simulink model "PV_MODEL"  (R2024b)
settings: Solver=ode23t  StartTime=0.0  StopTime=2.4  FixedStep=1e-6  RelTol=1e-3
libraries: spsSeriesRLCBranchLib x12, spsFirstOrderFilterLib x9, spsIGBTDiodeLib x7, slpidlib x5, simulink x5, spsThreePhaseVIMeasurementLib x2, spsabctodq0Lib x2, spsAlphaBetaZerotodq0Lib x1, spsDiodeLib x1, spsPVArrayLib x1, spsPower3phInstantaneousLib x1, spsThreePhaseSourceLib x1
settings Model: Creator=Baymax  LastModifiedBy=Baymax

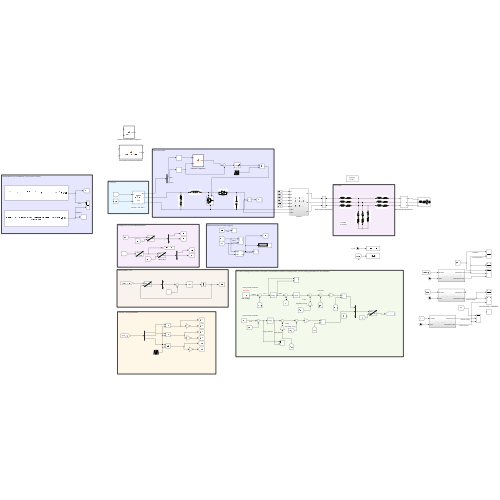
[thumbnail: Simulink's stored preview of the top-level diagram]
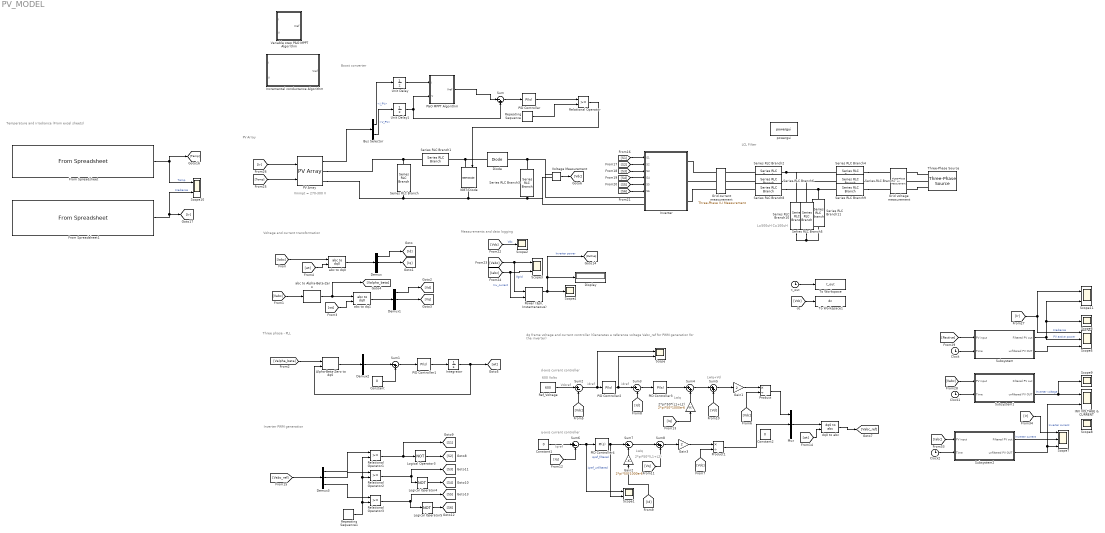
== system PV_MODEL ==
  note: Measurements and data logging
  note: Vmmpt = 270-300 V
  note: PV Array
  note: Boost converter
  note: L=500uH
      | C=100uH
  note: LCL Filter
  note: Inverter PWM generation
  note: dq frame voltage and current controller (Generates a reference voltage Vabc_ref for PWM generation for the inverter)
  note: Three phase - PLL
  note: Voltage and current transformation
  note: d-axis current controller
  note: LwIq+Vd
  note: 600 Volts
  note: 2*pi*50*(L1+L2)
  note: Vdcref
  note: idref
  note: q-axis current controller
  note: LwIq
  note: Iqref
  note: LwIq
  note: idref
  note: Temperature and irradiance (From excel sheets)
  2*pi*50*(L1+L2) : Gain  Gain=2*pi*50*1000e-6
  Alpha-Beta-Zero to dq0 : spsAlphaBetaZerotodq0Lib/Alpha-Beta-Zero to dq0  Alignment=90 degrees behind phase A axis
  Bus Selector : BusSelector  OutputSignals=I_PV,V_PV
  Clock : Clock
  Clock1 : Clock
  Clock2 : Clock
  Constant : Constant  Value=0
  Constant1 : Constant  Value=0
  Constant2 : Constant  Value=0
  Demux{,1..3} (4 alike) : Demux  Outputs=3
  Diode : spsDiodeLib/Diode  Ron=0.001  Lon=0  Vf=0.8  IC=0  UseSnubber=0  Rs=500  Cs=250e-9  Measurements=off
  Display : Display
  From Spreadsheet : FromSpreadsheet  FileName=C:\Users\Baymax\Desktop\Mr.Usamah\Profiles\granular\temperature_profile.xlsx  SheetName=temperature_profile  Range=A2:B2002
  From Spreadsheet1 : FromSpreadsheet  FileName=C:\Users\Baymax\Desktop\Mr.Usamah\Profiles\granular\Irradiance_profile_granular.xlsx  SheetName=irradiance_data  Range=A2:B2002
  Gain1 : Gain  Gain=2
  Gain2 : Gain  Gain=2*pi*50*1000e-6
  Gain3 : Gain  Gain=2
  Grid current measurement : spsThreePhaseVIMeasurementLib/Three-Phase V-I Measurement  VoltageMeasurement=no  SetLabelV=off  LabelV=Vabc  Vpu=off  VpuLL=off  CurrentMeasurement=yes  SetLabelI=on  LabelI=Iabc  Ipu=off  Pbase=100e6  Vbase=500e3  OutputType=Complex  PhasorSimulation=off  PSBequivalent=0
  Grid voltage measurement : spsThreePhaseVIMeasurementLib/Three-Phase V-I Measurement  VoltageMeasurement=phase-to-ground  SetLabelV=on  LabelV=Vabc  Vpu=off  VpuLL=off  CurrentMeasurement=no  SetLabelI=on  LabelI=Iabc  Ipu=off  Pbase=100e6  Vbase=500e3  OutputType=Complex  PhasorSimulation=off  PSBequivalent=0
  IGBT/Diode : spsIGBTDiodeLib/IGBT//Diode  Ron=1e-3  Rs=1e5  Cs=inf  Measurements=off
  INV VOLTAGE & CURRENT : Scope  NumInputPorts=2
  Incremental conductance Algorithm : MATLAB Function  TreatAsAtomicUnit=on
  Integrator : Integrator
  "Inverter " : Subsystem
  Logical Operator3 : Logic  Operator=NOT  IconShape=distinctive  AllPortsSameDT=off  OutDataTypeStr=boolean
  Logical Operator4 : Logic  Operator=NOT  IconShape=distinctive  AllPortsSameDT=off  OutDataTypeStr=boolean
  Logical Operator5 : Logic  Operator=NOT  IconShape=distinctive  AllPortsSameDT=off  OutDataTypeStr=boolean
  Mux : Mux  Inputs=3
  P&O MPPT Algorithm : MATLAB Function  TreatAsAtomicUnit=on
  PID Controller : slpidlib/PID Controller  Controller=PI  Form=Parallel  TimeDomain=Continuous-time  UseExternalTs=off  SampleTime=-1  IntegratorMethod=Forward Euler  FilterMethod=Forward Euler  ControllerParametersSource=internal  P=0.05  I=0.01  UseKiTs=off  D=0  UseExternalDerivativeSource=off  N=100  UseFilter=on  TunerSelectOption=Transfer Function Based (PID Tuner App)  InitialConditionSource=internal  InitialConditionForIntegrator=0  InitialConditionForFilter=0  DifferentiatorICPrevScaledInput=0  ExternalReset=none  TrackingMode=off  Kt=1  LimitOutput=on  SatLimitsSource=internal  UpperSaturationLimit=0.95  LowerSaturationLimit=0  LinearizeAsGain=on  AntiWindupMode=none  Kb=1  LimitIntegrator=off  UpperIntegratorSaturationLimit=inf  LowerIntegratorSaturationLimit=-inf  POutMin=[]  POutMax=[]  IOutMin=[]  IOutMax=[]  DOutMin=[]  DOutMax=[]  NOutMin=[]  NOutMax=[]  SumOutMin=[]  SumOutMax=[]  SaturationOutMin=[]  SaturationOutMax=[]  PParamMin=[]  PParamMax=[]  IParamMin=[]  IParamMax=[]  DParamMin=[]  DParamMax=[]  NParamMin=[]  NParamMax=[]  KbParamMin=[]  KbParamMax=[]  KtParamMin=[]  KtParamMax=[]  KbOutMin=[]  KbOutMax=[]  KtOutMin=[]  KtOutMax=[]  IntegratorOutMin=[]  IntegratorOutMax=[]  FilterOutMin=[]  FilterOutMax=[]  SumI1OutMin=[]  SumI1OutMax=[]  SumI2OutMin=[]  SumI2OutMax=[]  SumI3OutMin=[]  SumI3OutMax=[]  SumI4OutMin=[]  SumI4OutMax=[]  SumDOutMin=[]  SumDOutMax=[]  DifferentiatorOutMin=[]  DifferentiatorOutMax=[]  FilterDiffOutCoefMin=[]  FilterDiffOutCoefMax=[]  ReciprocalOutMin=[]  ReciprocalOutMax=[]  SumDenOutMin=[]  SumDenOutMax=[]  SumNumOutMin=[]  SumNumOutMax=[]  DivideOutMin=[]  DivideOutMax=[]  UdiffTsProdOutMin=[]  UdiffTsProdOutMax=[]  NTsProdOutMin=[]  NTsProdOutMax=[]  UintegralTsProdOutMin=[]  UintegralTsProdOutMax=[]  UngainTsProdOutMin=[]  UngainTsProdOutMax=[]  ClampingZeroOutDataTypeStr=Inherit: Inherit via back propagation  ClampingZeroOutMin=[]  ClampingZeroOutMax=[]  FilterDenConstantOutDataTypeStr=Inherit: Inherit via back propagation  FilterDenConstantOutMin=[]  FilterDenConstantOutMax=[]  PCopyOutDataTypeStr=Inherit: Inherit via back propagation  PCopyOutMin=[]  PCopyOutMax=[]  NCopyOutDataTypeStr=Inherit: Inherit via back propagation  NCopyOutMin=[]  NCopyOutMax=[]  IntegratorContinuousStateAttributes=''  IntegratorStateMustResolveToSignalObject=off  IntegratorRTWStateStorageClass=Auto  FilterContinuousStateAttributes=''  FilterStateMustResolveToSignalObject=off  FilterRTWStateStorageClass=Auto  ParallelPVariant=InternalParameters  IdealPVariant=Disabled  IVariant=InternalParameters  DVariant=Disabled  IntegratorVariant=Continuous  SatVariant=Enabled  AWVariant=Passthrough  PCopyVariant=Disabled  TRVariant=Disabled  FdbkBlocksVariant=Forward  IdealPFdbkVariant=Disabled  SatFdbkVariant=Disabled  DerivativeFilterVariant=Disabled  NVariant=Disabled  NCopyVariant=Disabled_SignalSpec  FilterICVariant=Disabled  IntegratorICVariant=InternalICs  ExternalResetVariant=Disabled  TRSumVariant=Passthrough  SumFdbkVariant=Disabled  SumVariant=Sum_PI  TsampFilterVariant=InternalTs  TsampNgainVariant=Passthrough  TsampIntegralVariant=Disabled_SignalSpec  ExternalSaturationOutDataTypeStr=Inherit: Same as second input  DerivativeSourceVariant=Disabled  PreIntVariant=InternalPreInt
  PID Controller1 : slpidlib/PID Controller  Controller=PI  Form=Parallel  TimeDomain=Continuous-time  UseExternalTs=off  SampleTime=-1  IntegratorMethod=Forward Euler  FilterMethod=Forward Euler  ControllerParametersSource=internal  P=10  I=50000  UseKiTs=off  D=0  UseExternalDerivativeSource=off  N=100  UseFilter=on  TunerSelectOption=Transfer Function Based (PID Tuner App)  InitialConditionSource=internal  InitialConditionForIntegrator=0  InitialConditionForFilter=0  DifferentiatorICPrevScaledInput=0  ExternalReset=none  TrackingMode=off  Kt=1  LimitOutput=off  SatLimitsSource=internal  UpperSaturationLimit=inf  LowerSaturationLimit=-inf  LinearizeAsGain=on  AntiWindupMode=none  Kb=1  LimitIntegrator=off  UpperIntegratorSaturationLimit=inf  LowerIntegratorSaturationLimit=-inf  POutMin=[]  POutMax=[]  IOutMin=[]  IOutMax=[]  DOutMin=[]  DOutMax=[]  NOutMin=[]  NOutMax=[]  SumOutMin=[]  SumOutMax=[]  SaturationOutMin=[]  SaturationOutMax=[]  PParamMin=[]  PParamMax=[]  IParamMin=[]  IParamMax=[]  DParamMin=[]  DParamMax=[]  NParamMin=[]  NParamMax=[]  KbParamMin=[]  KbParamMax=[]  KtParamMin=[]  KtParamMax=[]  KbOutMin=[]  KbOutMax=[]  KtOutMin=[]  KtOutMax=[]  IntegratorOutMin=[]  IntegratorOutMax=[]  FilterOutMin=[]  FilterOutMax=[]  SumI1OutMin=[]  SumI1OutMax=[]  SumI2OutMin=[]  SumI2OutMax=[]  SumI3OutMin=[]  SumI3OutMax=[]  SumI4OutMin=[]  SumI4OutMax=[]  SumDOutMin=[]  SumDOutMax=[]  DifferentiatorOutMin=[]  DifferentiatorOutMax=[]  FilterDiffOutCoefMin=[]  FilterDiffOutCoefMax=[]  ReciprocalOutMin=[]  ReciprocalOutMax=[]  SumDenOutMin=[]  SumDenOutMax=[]  SumNumOutMin=[]  SumNumOutMax=[]  DivideOutMin=[]  DivideOutMax=[]  UdiffTsProdOutMin=[]  UdiffTsProdOutMax=[]  NTsProdOutMin=[]  NTsProdOutMax=[]  UintegralTsProdOutMin=[]  UintegralTsProdOutMax=[]  UngainTsProdOutMin=[]  UngainTsProdOutMax=[]  ClampingZeroOutDataTypeStr=Inherit: Inherit via back propagation  ClampingZeroOutMin=[]  ClampingZeroOutMax=[]  FilterDenConstantOutDataTypeStr=Inherit: Inherit via back propagation  FilterDenConstantOutMin=[]  FilterDenConstantOutMax=[]  PCopyOutDataTypeStr=Inherit: Inherit via back propagation  PCopyOutMin=[]  PCopyOutMax=[]  NCopyOutDataTypeStr=Inherit: Inherit via back propagation  NCopyOutMin=[]  NCopyOutMax=[]  IntegratorContinuousStateAttributes=''  IntegratorStateMustResolveToSignalObject=off  IntegratorRTWStateStorageClass=Auto  FilterContinuousStateAttributes=''  FilterStateMustResolveToSignalObject=off  FilterRTWStateStorageClass=Auto  ParallelPVariant=InternalParameters  IdealPVariant=Disabled  IVariant=InternalParameters  DVariant=Disabled  IntegratorVariant=Continuous  SatVariant=Disabled  AWVariant=Passthrough  PCopyVariant=Disabled  TRVariant=Disabled  FdbkBlocksVariant=Forward  IdealPFdbkVariant=Disabled  SatFdbkVariant=Disabled  DerivativeFilterVariant=Disabled  NVariant=Disabled  NCopyVariant=Disabled_SignalSpec  FilterICVariant=Disabled  IntegratorICVariant=InternalICs  ExternalResetVariant=Disabled  TRSumVariant=Passthrough  SumFdbkVariant=Disabled  SumVariant=Sum_PI  TsampFilterVariant=InternalTs  TsampNgainVariant=Passthrough  TsampIntegralVariant=Disabled_SignalSpec  ExternalSaturationOutDataTypeStr=Inherit: Same as second input  DerivativeSourceVariant=Disabled  PreIntVariant=InternalPreInt
  PID Controller2 : slpidlib/PID Controller  Controller=PI  Form=Parallel  TimeDomain=Continuous-time  UseExternalTs=off  SampleTime=-1  IntegratorMethod=Forward Euler  FilterMethod=Forward Euler  ControllerParametersSource=internal  P=0.25  I=300  UseKiTs=off  D=0  UseExternalDerivativeSource=off  N=100  UseFilter=on  TunerSelectOption=Transfer Function Based (PID Tuner App)  InitialConditionSource=internal  InitialConditionForIntegrator=0  InitialConditionForFilter=0  DifferentiatorICPrevScaledInput=0  ExternalReset=none  TrackingMode=off  Kt=1  LimitOutput=off  SatLimitsSource=internal  UpperSaturationLimit=inf  LowerSaturationLimit=-inf  LinearizeAsGain=on  AntiWindupMode=none  Kb=1  LimitIntegrator=off  UpperIntegratorSaturationLimit=inf  LowerIntegratorSaturationLimit=-inf  POutMin=[]  POutMax=[]  IOutMin=[]  IOutMax=[]  DOutMin=[]  DOutMax=[]  NOutMin=[]  NOutMax=[]  SumOutMin=[]  SumOutMax=[]  SaturationOutMin=[]  SaturationOutMax=[]  PParamMin=[]  PParamMax=[]  IParamMin=[]  IParamMax=[]  DParamMin=[]  DParamMax=[]  NParamMin=[]  NParamMax=[]  KbParamMin=[]  KbParamMax=[]  KtParamMin=[]  KtParamMax=[]  KbOutMin=[]  KbOutMax=[]  KtOutMin=[]  KtOutMax=[]  IntegratorOutMin=[]  IntegratorOutMax=[]  FilterOutMin=[]  FilterOutMax=[]  SumI1OutMin=[]  SumI1OutMax=[]  SumI2OutMin=[]  SumI2OutMax=[]  SumI3OutMin=[]  SumI3OutMax=[]  SumI4OutMin=[]  SumI4OutMax=[]  SumDOutMin=[]  SumDOutMax=[]  DifferentiatorOutMin=[]  DifferentiatorOutMax=[]  FilterDiffOutCoefMin=[]  FilterDiffOutCoefMax=[]  ReciprocalOutMin=[]  ReciprocalOutMax=[]  SumDenOutMin=[]  SumDenOutMax=[]  SumNumOutMin=[]  SumNumOutMax=[]  DivideOutMin=[]  DivideOutMax=[]  UdiffTsProdOutMin=[]  UdiffTsProdOutMax=[]  NTsProdOutMin=[]  NTsProdOutMax=[]  UintegralTsProdOutMin=[]  UintegralTsProdOutMax=[]  UngainTsProdOutMin=[]  UngainTsProdOutMax=[]  ClampingZeroOutDataTypeStr=Inherit: Inherit via back propagation  ClampingZeroOutMin=[]  ClampingZeroOutMax=[]  FilterDenConstantOutDataTypeStr=Inherit: Inherit via back propagation  FilterDenConstantOutMin=[]  FilterDenConstantOutMax=[]  PCopyOutDataTypeStr=Inherit: Inherit via back propagation  PCopyOutMin=[]  PCopyOutMax=[]  NCopyOutDataTypeStr=Inherit: Inherit via back propagation  NCopyOutMin=[]  NCopyOutMax=[]  IntegratorContinuousStateAttributes=''  IntegratorStateMustResolveToSignalObject=off  IntegratorRTWStateStorageClass=Auto  FilterContinuousStateAttributes=''  FilterStateMustResolveToSignalObject=off  FilterRTWStateStorageClass=Auto  ParallelPVariant=InternalParameters  IdealPVariant=Disabled  IVariant=InternalParameters  DVariant=Disabled  IntegratorVariant=Continuous  SatVariant=Disabled  AWVariant=Passthrough  PCopyVariant=Disabled  TRVariant=Disabled  FdbkBlocksVariant=Forward  IdealPFdbkVariant=Disabled  SatFdbkVariant=Disabled  DerivativeFilterVariant=Disabled  NVariant=Disabled  NCopyVariant=Disabled_SignalSpec  FilterICVariant=Disabled  IntegratorICVariant=InternalICs  ExternalResetVariant=Disabled  TRSumVariant=Passthrough  SumFdbkVariant=Disabled  SumVariant=Sum_PI  TsampFilterVariant=InternalTs  TsampNgainVariant=Passthrough  TsampIntegralVariant=Disabled_SignalSpec  ExternalSaturationOutDataTypeStr=Inherit: Same as second input  DerivativeSourceVariant=Disabled  PreIntVariant=InternalPreInt
  PID Controller3 : slpidlib/PID Controller  Controller=PI  Form=Parallel  TimeDomain=Continuous-time  UseExternalTs=off  SampleTime=-1  IntegratorMethod=Forward Euler  FilterMethod=Forward Euler  ControllerParametersSource=internal  P=10  I=20  UseKiTs=off  D=0  UseExternalDerivativeSource=off  N=100  UseFilter=on  TunerSelectOption=Transfer Function Based (PID Tuner App)  InitialConditionSource=internal  InitialConditionForIntegrator=0  InitialConditionForFilter=0  DifferentiatorICPrevScaledInput=0  ExternalReset=none  TrackingMode=off  Kt=1  LimitOutput=off  SatLimitsSource=internal  UpperSaturationLimit=inf  LowerSaturationLimit=-inf  LinearizeAsGain=on  AntiWindupMode=none  Kb=1  LimitIntegrator=off  UpperIntegratorSaturationLimit=inf  LowerIntegratorSaturationLimit=-inf  POutMin=[]  POutMax=[]  IOutMin=[]  IOutMax=[]  DOutMin=[]  DOutMax=[]  NOutMin=[]  NOutMax=[]  SumOutMin=[]  SumOutMax=[]  SaturationOutMin=[]  SaturationOutMax=[]  PParamMin=[]  PParamMax=[]  IParamMin=[]  IParamMax=[]  DParamMin=[]  DParamMax=[]  NParamMin=[]  NParamMax=[]  KbParamMin=[]  KbParamMax=[]  KtParamMin=[]  KtParamMax=[]  KbOutMin=[]  KbOutMax=[]  KtOutMin=[]  KtOutMax=[]  IntegratorOutMin=[]  IntegratorOutMax=[]  FilterOutMin=[]  FilterOutMax=[]  SumI1OutMin=[]  SumI1OutMax=[]  SumI2OutMin=[]  SumI2OutMax=[]  SumI3OutMin=[]  SumI3OutMax=[]  SumI4OutMin=[]  SumI4OutMax=[]  SumDOutMin=[]  SumDOutMax=[]  DifferentiatorOutMin=[]  DifferentiatorOutMax=[]  FilterDiffOutCoefMin=[]  FilterDiffOutCoefMax=[]  ReciprocalOutMin=[]  ReciprocalOutMax=[]  SumDenOutMin=[]  SumDenOutMax=[]  SumNumOutMin=[]  SumNumOutMax=[]  DivideOutMin=[]  DivideOutMax=[]  UdiffTsProdOutMin=[]  UdiffTsProdOutMax=[]  NTsProdOutMin=[]  NTsProdOutMax=[]  UintegralTsProdOutMin=[]  UintegralTsProdOutMax=[]  UngainTsProdOutMin=[]  UngainTsProdOutMax=[]  ClampingZeroOutDataTypeStr=Inherit: Inherit via back propagation  ClampingZeroOutMin=[]  ClampingZeroOutMax=[]  FilterDenConstantOutDataTypeStr=Inherit: Inherit via back propagation  FilterDenConstantOutMin=[]  FilterDenConstantOutMax=[]  PCopyOutDataTypeStr=Inherit: Inherit via back propagation  PCopyOutMin=[]  PCopyOutMax=[]  NCopyOutDataTypeStr=Inherit: Inherit via back propagation  NCopyOutMin=[]  NCopyOutMax=[]  IntegratorContinuousStateAttributes=''  IntegratorStateMustResolveToSignalObject=off  IntegratorRTWStateStorageClass=Auto  FilterContinuousStateAttributes=''  FilterStateMustResolveToSignalObject=off  FilterRTWStateStorageClass=Auto  ParallelPVariant=InternalParameters  IdealPVariant=Disabled  IVariant=InternalParameters  DVariant=Disabled  IntegratorVariant=Continuous  SatVariant=Disabled  AWVariant=Passthrough  PCopyVariant=Disabled  TRVariant=Disabled  FdbkBlocksVariant=Forward  IdealPFdbkVariant=Disabled  SatFdbkVariant=Disabled  DerivativeFilterVariant=Disabled  NVariant=Disabled  NCopyVariant=Disabled_SignalSpec  FilterICVariant=Disabled  IntegratorICVariant=InternalICs  ExternalResetVariant=Disabled  TRSumVariant=Passthrough  SumFdbkVariant=Disabled  SumVariant=Sum_PI  TsampFilterVariant=InternalTs  TsampNgainVariant=Passthrough  TsampIntegralVariant=Disabled_SignalSpec  ExternalSaturationOutDataTypeStr=Inherit: Same as second input  DerivativeSourceVariant=Disabled  PreIntVariant=InternalPreInt
  PID Controller4 : slpidlib/PID Controller  Controller=PI  Form=Parallel  TimeDomain=Continuous-time  UseExternalTs=off  SampleTime=-1  IntegratorMethod=Forward Euler  FilterMethod=Forward Euler  ControllerParametersSource=internal  P=10  I=20  UseKiTs=off  D=0  UseExternalDerivativeSource=off  N=100  UseFilter=on  TunerSelectOption=Transfer Function Based (PID Tuner App)  InitialConditionSource=internal  InitialConditionForIntegrator=0  InitialConditionForFilter=0  DifferentiatorICPrevScaledInput=0  ExternalReset=none  TrackingMode=off  Kt=1  LimitOutput=off  SatLimitsSource=internal  UpperSaturationLimit=inf  LowerSaturationLimit=-inf  LinearizeAsGain=on  AntiWindupMode=none  Kb=1  LimitIntegrator=off  UpperIntegratorSaturationLimit=inf  LowerIntegratorSaturationLimit=-inf  POutMin=[]  POutMax=[]  IOutMin=[]  IOutMax=[]  DOutMin=[]  DOutMax=[]  NOutMin=[]  NOutMax=[]  SumOutMin=[]  SumOutMax=[]  SaturationOutMin=[]  SaturationOutMax=[]  PParamMin=[]  PParamMax=[]  IParamMin=[]  IParamMax=[]  DParamMin=[]  DParamMax=[]  NParamMin=[]  NParamMax=[]  KbParamMin=[]  KbParamMax=[]  KtParamMin=[]  KtParamMax=[]  KbOutMin=[]  KbOutMax=[]  KtOutMin=[]  KtOutMax=[]  IntegratorOutMin=[]  IntegratorOutMax=[]  FilterOutMin=[]  FilterOutMax=[]  SumI1OutMin=[]  SumI1OutMax=[]  SumI2OutMin=[]  SumI2OutMax=[]  SumI3OutMin=[]  SumI3OutMax=[]  SumI4OutMin=[]  SumI4OutMax=[]  SumDOutMin=[]  SumDOutMax=[]  DifferentiatorOutMin=[]  DifferentiatorOutMax=[]  FilterDiffOutCoefMin=[]  FilterDiffOutCoefMax=[]  ReciprocalOutMin=[]  ReciprocalOutMax=[]  SumDenOutMin=[]  SumDenOutMax=[]  SumNumOutMin=[]  SumNumOutMax=[]  DivideOutMin=[]  DivideOutMax=[]  UdiffTsProdOutMin=[]  UdiffTsProdOutMax=[]  NTsProdOutMin=[]  NTsProdOutMax=[]  UintegralTsProdOutMin=[]  UintegralTsProdOutMax=[]  UngainTsProdOutMin=[]  UngainTsProdOutMax=[]  ClampingZeroOutDataTypeStr=Inherit: Inherit via back propagation  ClampingZeroOutMin=[]  ClampingZeroOutMax=[]  FilterDenConstantOutDataTypeStr=Inherit: Inherit via back propagation  FilterDenConstantOutMin=[]  FilterDenConstantOutMax=[]  PCopyOutDataTypeStr=Inherit: Inherit via back propagation  PCopyOutMin=[]  PCopyOutMax=[]  NCopyOutDataTypeStr=Inherit: Inherit via back propagation  NCopyOutMin=[]  NCopyOutMax=[]  IntegratorContinuousStateAttributes=''  IntegratorStateMustResolveToSignalObject=off  IntegratorRTWStateStorageClass=Auto  FilterContinuousStateAttributes=''  FilterStateMustResolveToSignalObject=off  FilterRTWStateStorageClass=Auto  ParallelPVariant=InternalParameters  IdealPVariant=Disabled  IVariant=InternalParameters  DVariant=Disabled  IntegratorVariant=Continuous  SatVariant=Disabled  AWVariant=Passthrough  PCopyVariant=Disabled  TRVariant=Disabled  FdbkBlocksVariant=Forward  IdealPFdbkVariant=Disabled  SatFdbkVariant=Disabled  DerivativeFilterVariant=Disabled  NVariant=Disabled  NCopyVariant=Disabled_SignalSpec  FilterICVariant=Disabled  IntegratorICVariant=InternalICs  ExternalResetVariant=Disabled  TRSumVariant=Passthrough  SumFdbkVariant=Disabled  SumVariant=Sum_PI  TsampFilterVariant=InternalTs  TsampNgainVariant=Passthrough  TsampIntegralVariant=Disabled_SignalSpec  ExternalSaturationOutDataTypeStr=Inherit: Same as second input  DerivativeSourceVariant=Disabled  PreIntVariant=InternalPreInt
  PV Array : spsPVArrayLib/PV Array  Npar=47  Nser=10  PlotType=array @ 1000 W/m2 & specified temperatures  S_vec="[ 1000  500  100 ]"  Temp_C_vec="[ 45 25  ]"  ModuleName=A10Green Technology A10J-M60-220  PlotWhenSelected=off  Pm=219.876  Ncell=60  Voc=36.06  Isc=7.95  Vm=30.12  Im=7.3  beta_Voc_pc=-0.3624  alpha_Isc_pc=0.054805  beta_Voc=-0.13068  alpha_Isc=0.004357  IL=7.9642  I0=2.8692e-10  nI=0.97455  Rsh=106.1817  Rs=0.18964  RobustModel=off  RobustCellTemperature=313.3991  BAL=on  Tc=1e-6  Tfilter=5e-5
  "Power (3ph, Instantaneous)" : spsPower3phInstantaneousLib/Power (3ph, Instantaneous)
  Product : Product  Inputs=*/
  Product1 : Product  Inputs=*/
  Ref_Voltage : Constant  Value=600
  Relational Operator{,1..3} (4 alike) : RelationalOperator  OutDataTypeStr=boolean  RndMeth=Simplest  InputSameDT=off
  Repeating Sequence : simulink/Sources/Repeating Sequence  rep_seq_t=[0 0.0002]  rep_seq_y=[0 1]
  Repeating Sequence1 : simulink/Sources/Repeating Sequence  rep_seq_t=[0 0.00005 0.0001]  rep_seq_y=[-1 1 -1]
  Scope{,1,3,10..11} (5 alike) : Scope  NumInputPorts=2
  Scope{2,4,6,8..9} (5 alike) : Scope
  Scope5 : Scope  NumInputPorts=3
  Scope7 : Scope  NumInputPorts=3
  Series RLC Branch : spsSeriesRLCBranchLib/Series RLC Branch  LConnTagsString=__new0  RConnTagsString=__new0  BranchType=RC  Resistance=1e-3  Inductance=1e-3  SetiL0=off  InitialCurrent=0  Capacitance=1000e-6  Setx0=off  InitialVoltage=0  Measurements=None
  Series RLC Branch1 : spsSeriesRLCBranchLib/Series RLC Branch  LConnTagsString=__new0  RConnTagsString=__new0  BranchType=L  Resistance=1  Inductance=1.45e-3  SetiL0=off  InitialCurrent=0  Capacitance=1e-6  Setx0=off  InitialVoltage=0  Measurements=None
  Series RLC Branch10 : spsSeriesRLCBranchLib/Series RLC Branch  LConnTagsString=__new0  RConnTagsString=__new0  BranchType=RC  Resistance=1e-3  Inductance=1e-3  SetiL0=off  InitialCurrent=0  Capacitance=100e-6  Setx0=off  InitialVoltage=0  Measurements=None
  Series RLC Branch11 : spsSeriesRLCBranchLib/Series RLC Branch  LConnTagsString=__new0  RConnTagsString=__new0  BranchType=RC  Resistance=1e-3  Inductance=1e-3  SetiL0=off  InitialCurrent=0  Capacitance=100e-6  Setx0=off  InitialVoltage=0  Measurements=None
  Series RLC Branch{2,4,6..9} (6 alike) : spsSeriesRLCBranchLib/Series RLC Branch  LConnTagsString=__new0  RConnTagsString=__new0  BranchType=RL  Resistance=1e-3  Inductance=500e-6  SetiL0=off  InitialCurrent=0  Capacitance=1e-6  Setx0=off  InitialVoltage=0  Measurements=None
  Series RLC Branch3 : spsSeriesRLCBranchLib/Series RLC Branch  LConnTagsString=__new0  RConnTagsString=__new0  BranchType=C  Resistance=1  Inductance=1e-3  SetiL0=off  InitialCurrent=0  Capacitance=3227e-6  Setx0=off  InitialVoltage=0  Measurements=None
  Series RLC Branch5 : spsSeriesRLCBranchLib/Series RLC Branch  LConnTagsString=__new0  RConnTagsString=__new0  BranchType=RC  Resistance=1e-3  Inductance=1e-3  SetiL0=off  InitialCurrent=0  Capacitance=100e-6  Setx0=off  InitialVoltage=0  Measurements=None
  Subsystem : Subsystem
  Subsystem1 : Subsystem
  Subsystem2 : Subsystem
  Sum : Sum  Inputs=|-+
  Sum1 : Sum  Inputs=|-+
  Sum{2..3,6..7} (4 alike) : Sum  Inputs=|+-
  Sum4 : Sum  Inputs=|++
  Sum5 : Sum  Inputs=|++
  Sum8 : Sum  Inputs=|++
  Three-Phase Source : spsThreePhaseSourceLib/Three-Phase Source  InternalConnection=Yg  VoltagePhases=off  Voltage=400  PhaseAngle=0  Voltage_phases=[25e3 25e3 25e3]/sqrt(3)  PhaseAngles_phases=[0 -120 +120]  Frequency=50  NonIdealSource=on  SpecifyImpedance=off  Resistance=1e-6  Inductance=1e-6  ShortCircuitLevel=100e6  BaseVoltage=400  XRratio=7  BusType=swing  Pref=10e3  Qref=0  Prefabc=[10e3, 10e3, 10e3]  Qrefabc=[0, 0, 0]  Qmin=-inf  Qmax=inf
  To Workspace : ToWorkspace  VariableName=t_out  SampleTime=-1
      settings: Decimation=5
  To Workspace1 : ToWorkspace  VariableName=dc  SampleTime=-1
      settings: Decimation=2
  Unit Delay : UnitDelay  SampleTime=1e-4  HasFrameUpgradeWarning=on
  Unit Delay1 : UnitDelay  SampleTime=1e-4  HasFrameUpgradeWarning=on
  Variable step P&O MPPT Algorithm : MATLAB Function  TreatAsAtomicUnit=on
  Voltage Measurement : spsVoltageMeasurementLib/Voltage Measurement  PhasorSimulation=off  OutputType=Complex  PSBequivalent=0
  abc to Alpha-Beta-Zero : spsabctoAlphaBetaZeroLib/abc to Alpha-Beta-Zero
  abc to dq0 : spsabctodq0Lib/abc to dq0  Alignment=90 degrees behind phase A axis
  abc to dq1 : spsabctodq0Lib/abc to dq0  Alignment=90 degrees behind phase A axis
  dq0 to abc : spsdq0toabcLib/dq0 to abc  Alignment=90 degrees behind phase A axis
  powergui : spspowerguiLib/powergui  Priority=1  SimulationMode=Discrete  SampleTime=1e-6  frequency=60  Iterations=50  frequencyindice=0  Pbase=100e6  ErrMax=1e-4  UnitsV=kV  UnitsW=MW  buscounter=0  FunctionMessages=off  echomessages=off  EnableUseOfTLC=off  CurrentSourceSwitches=off  DisableSnubberDevices=off  DisableRonSwitches=off  DisableVfSwitches=off  DisplayEquations=off  AutomaticDiscreteSolvers=off  SolverType=Tustin/Backward Euler (TBE)  Interpol=off  ExternalGateDelay=off  methode=off  Ts=100  x0status=blocks  SPID=on  SwTol=0  HookPort=off  NonlinearTolerance=1e-4  nMaxIteration=100  ContinueOnMaxIteration=off  RestoreLinks=warning  ResistiveCurrentMeasurement=off  Frange=[0:2:500]  Ylog=off  Xlog=on  ShowGrid=off  save=off  variable=ZData  structure=0  ZoomFFT=off  StartTime=0.0  cycles=1  DisplayStyle=1  fundamental=60  FreqAxis=off  MaxFrequency=1000  frequencyindicesteady=1  RmsSteady=1  display=off
  t_out : Clock
  wires:
  PV Array/1 -> Bus Selector/1
  Bus Selector/1 -> Unit Delay/1  "<I_PV>"
  Bus Selector/2 -> Unit Delay1/1  "<V_PV>"
  Unit Delay1/1 -> P&O MPPT Algorithm/2(V), Sum/2
  Sum/1 -> PID Controller/1
  PID Controller/1 -> Relational Operator/1
  Repeating Sequence/1 -> Relational Operator/2
  Relational Operator/1 -> IGBT/Diode/1
  [Iabc] -> abc to dq0/1
  abc to dq0/1 -> Demux/1
  Demux/1 -> [Id]
  Demux/2 -> [Iq]
  [Vabc] -> abc to Alpha-Beta-Zero/1
  abc to Alpha-Beta-Zero/1 -> [Valpha_beta], abc to dq1/1
  Demux1/2 -> [Vq]
  Demux1/1 -> [Vd]
  abc to dq1/1 -> Demux1/1
  [Valpha_beta] -> Alpha-Beta-Zero to dq0/1
  Alpha-Beta-Zero to dq0/1 -> Demux2/1
  Demux2/2 -> Sum1/1
  Constant/1 -> Sum1/2
  Sum1/1 -> PID Controller1/1
  PID Controller1/1 -> Integrator/1
  Integrator/1 -> [wt], Alpha-Beta-Zero to dq0/2
  [wt] -> abc to dq1/2
  [wt] -> abc to dq0/2
  Gain2/1 -> Sum7/2
  2*pi*50*(L1+L2)/1 -> Sum4/2
  Sum6/1 -> Scope1/1, PID Controller4/1  "iqref_unfiltered"
  [Vq] -> Sum8/2
  PID Controller3/1 -> Sum4/1
  Product/1 -> Mux/1
  Constant1/1 -> Sum6/1
  Mux/1 -> dq0 to abc/1
  Ref_Voltage/1 -> Sum2/1
  Gain3/1 -> Product1/1
  Sum8/1 -> Gain3/1
  PID Controller4/1 -> Sum7/1, Scope1/2  "iqref_filtered"
  Sum4/1 -> Sum5/1
  Sum2/1 -> Scope/1, PID Controller2/1
  Sum3/1 -> PID Controller3/1
  Product1/1 -> Mux/2
  PID Controller2/1 -> Scope/2, Sum3/1
  [Vd] -> Sum5/2
  Sum7/1 -> Sum8/1
  Sum5/1 -> Gain1/1
  Gain1/1 -> Product/1
  Voltage Measurement/1 -> [Vdc]
  [Vdc] -> Sum2/2
  [Vdc] -> Product/2
  [Vdc] -> Product1/2
  [Id] -> Sum3/2
  [Id] -> Gain2/1
  [Iq] -> Sum6/2
  [Iq] -> 2*pi*50*(L1+L2)/1
  [wt] -> dq0 to abc/2
  dq0 to abc/1 -> [Vabc_ref]
  [Vabc_ref] -> Demux3/1
  Demux3/1 -> Relational Operator1/1
  Demux3/2 -> Relational Operator2/1
  Demux3/3 -> Relational Operator3/1
  Repeating Sequence1/1 -> Relational Operator3/2, Relational Operator2/2, Relational Operator1/2
  Relational Operator1/1 -> [S1], Logical Operator3/1
  Logical Operator3/1 -> [S2]
  Relational Operator2/1 -> Logical Operator4/1, [S3]
  Logical Operator4/1 -> [S4]
  Relational Operator3/1 -> Logical Operator5/1, [S5]
  Logical Operator5/1 -> [S6]
  [S1] -> "Inverter "/1(S1)
  [S2] -> "Inverter "/2(S2)
  [S3] -> "Inverter "/3(S3)
  [S4] -> "Inverter "/4(S4)
  [S5] -> "Inverter "/5(S5)
  [S6] -> "Inverter "/6(S6)
  [Vdc] -> Scope2/1  "Vdc"
  [Vabc] -> "Power (3ph, Instantaneous)"/1, Scope3/1  "Vgrid"
  [Iabc] -> "Power (3ph, Instantaneous)"/2, Scope3/2  "Inv_current"
  "Power (3ph, Instantaneous)"/1 -> [Pactive], Display/1, Scope4/1  "Inverter power"
  [Ir] -> PV Array/1
  [Temp] -> PV Array/2
  From Spreadsheet/1 -> [Temp], Scope10/1  "Temp"
  From Spreadsheet1/1 -> Scope10/2, [Ir]  "Irradiance"
  P&O MPPT Algorithm/1(Vref) -> Sum/1
  [Vdc] -> To Workspace1/1
  t_out/1 -> To Workspace/1
  Unit Delay/1 -> P&O MPPT Algorithm/1(I)
  Subsystem/2(unfiltered PV OUT) -> Scope5/3
  Subsystem/1(Filtered PV out) -> Scope11/2, Scope6/1, Scope5/2  "PV active power"
  [Ir] -> Scope5/1, Scope11/1  "Irradiance"
  [Pactive] -> Subsystem/1(PV input)
  Clock/1 -> Subsystem/2(Time)
  Clock1/1 -> Subsystem1/2(Time)
  [Vabc] -> Subsystem1/1(PV input)
  Subsystem1/2(unfiltered PV OUT) -> Scope9/1, INV VOLTAGE & CURRENT/1  "Inverter voltage"
  Subsystem2/2(unfiltered PV OUT) -> INV VOLTAGE & CURRENT/2, Scope7/3  "Inverter current"
  Subsystem2/1(Filtered PV out) -> Scope7/2  "Inverter current"
  [Ir] -> Scope7/1
  [Iabc] -> Subsystem2/1(PV input)
  Clock2/1 -> Subsystem2/2(Time)
  connections:
  Diode/LConn1 -- IGBT/Diode/LConn1 -- Series RLC Branch1/LConn1
  Series RLC Branch1/RConn1 -- PV Array/RConn1 -- Series RLC Branch/LConn1
  Series RLC Branch/RConn1 -- PV Array/RConn2 -- "Inverter "/LConn2 -- Voltage Measurement/LConn2 -- Series RLC Branch3/RConn1 -- IGBT/Diode/RConn1
  Series RLC Branch3/LConn1 -- Voltage Measurement/LConn1 -- "Inverter "/LConn1 -- Diode/RConn1
  Grid current measurement/LConn2 -- "Inverter "/RConn2
  Series RLC Branch2/RConn1 -- Grid current measurement/RConn1
  Series RLC Branch2/LConn1 -- Series RLC Branch10/RConn1 -- Series RLC Branch4/RConn1
  Three-Phase Source/RConn1 -- Grid voltage measurement/LConn1
  Three-Phase Source/RConn2 -- Grid voltage measurement/LConn2
  Three-Phase Source/RConn3 -- Grid voltage measurement/LConn3
  Series RLC Branch4/LConn1 -- Grid voltage measurement/RConn1
  Series RLC Branch6/RConn1 -- Grid current measurement/RConn2
  Series RLC Branch6/LConn1 -- Series RLC Branch5/RConn1 -- Series RLC Branch7/RConn1
  Series RLC Branch7/LConn1 -- Grid voltage measurement/RConn2
  Series RLC Branch8/RConn1 -- Grid current measurement/RConn3
  Series RLC Branch9/LConn1 -- Grid voltage measurement/RConn3
  Series RLC Branch11/RConn1 -- Series RLC Branch9/RConn1 -- Series RLC Branch8/LConn1
  Series RLC Branch11/LConn1 -- Series RLC Branch10/LConn1 -- Series RLC Branch5/LConn1
  Grid current measurement/LConn1 -- "Inverter "/RConn1
  Grid current measurement/LConn3 -- "Inverter "/RConn3

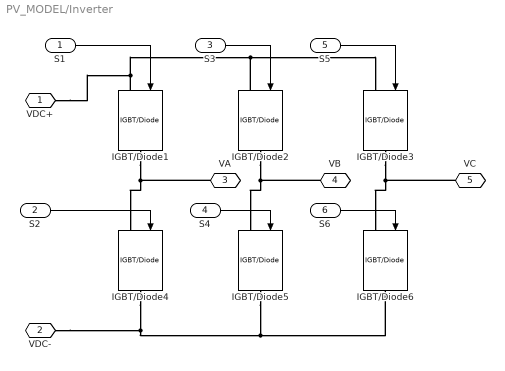
== system PV_MODEL/Inverter  ==
  S1 : Inport
  S2 : Inport  Port=2
  S3 : Inport  Port=3
  S4 : Inport  Port=4
  S5 : Inport  Port=5
  S6 : Inport  Port=6
  IGBT/Diode{1..6} (6 alike) : spsIGBTDiodeLib/IGBT//Diode  Ron=1e-3  Rs=1e5  Cs=inf  Measurements=off
  VDC+ : PMIOPort  Side=Left
  VDC- : PMIOPort  Port=2  Side=Left
  VA : PMIOPort  Port=3  Side=Right
  VB : PMIOPort  Port=4  Side=Right
  VC : PMIOPort  Port=5  Side=Right
  wires:
  S3/1 -> IGBT/Diode2/1
  S2/1 -> IGBT/Diode4/1
  S1/1 -> IGBT/Diode1/1
  S4/1 -> IGBT/Diode5/1
  S6/1 -> IGBT/Diode6/1
  S5/1 -> IGBT/Diode3/1
  connections:
  IGBT/Diode1/LConn1 -- VDC+/RConn1 -- IGBT/Diode2/LConn1 -- IGBT/Diode3/LConn1
  IGBT/Diode2/RConn1 -- VB/RConn1 -- IGBT/Diode5/LConn1
  IGBT/Diode4/RConn1 -- VDC-/RConn1 -- IGBT/Diode6/RConn1 -- IGBT/Diode5/RConn1
  IGBT/Diode1/RConn1 -- VA/RConn1 -- IGBT/Diode4/LConn1
  IGBT/Diode3/RConn1 -- VC/RConn1 -- IGBT/Diode6/LConn1

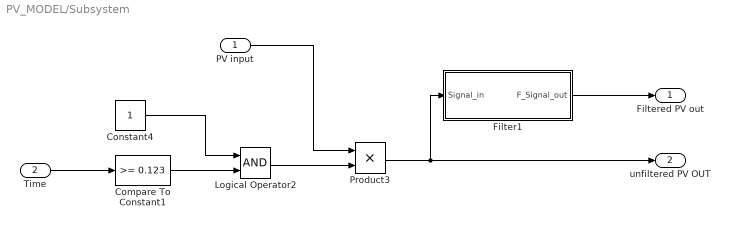
== system PV_MODEL/Subsystem ==
  PV input : Inport
  Time : Inport  Port=2
  Compare To Constant1 : simulink/Logic and Bit Operations/Compare To Constant  relop=>=  const=0.123  OutDataTypeStr=boolean
  Constant4 : Constant
  Filter1 : Subsystem
  Logical Operator2 : Logic  AllPortsSameDT=off  OutDataTypeStr=boolean
  Product3 : Product
  Filtered PV out : Outport
  unfiltered PV OUT : Outport  Port=2
  wires:
  Product3/1 -> unfiltered PV OUT/1, Filter1/1(Signal_in)
  Time/1 -> Compare To Constant1/1
  Constant4/1 -> Logical Operator2/1
  Filter1/1(F_Signal_out) -> Filtered PV out/1
  PV input/1 -> Product3/1
  Logical Operator2/1 -> Product3/2
  Compare To Constant1/1 -> Logical Operator2/2

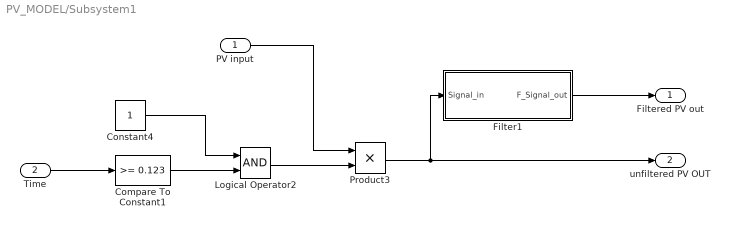
== system PV_MODEL/Subsystem1 ==
  PV input : Inport
  Time : Inport  Port=2
  Compare To Constant1 : simulink/Logic and Bit Operations/Compare To Constant  relop=>=  const=0.123  OutDataTypeStr=boolean
  Constant4 : Constant
  Filter1 : Subsystem
  Logical Operator2 : Logic  AllPortsSameDT=off  OutDataTypeStr=boolean
  Product3 : Product
  Filtered PV out : Outport
  unfiltered PV OUT : Outport  Port=2
  wires:
  Compare To Constant1/1 -> Logical Operator2/2
  Logical Operator2/1 -> Product3/2
  PV input/1 -> Product3/1
  Filter1/1(F_Signal_out) -> Filtered PV out/1
  Constant4/1 -> Logical Operator2/1
  Time/1 -> Compare To Constant1/1
  Product3/1 -> Filter1/1(Signal_in), unfiltered PV OUT/1

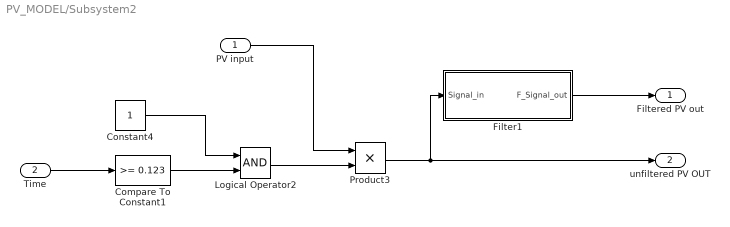
== system PV_MODEL/Subsystem2 ==
  PV input : Inport
  Time : Inport  Port=2
  Compare To Constant1 : simulink/Logic and Bit Operations/Compare To Constant  relop=>=  const=0.123  OutDataTypeStr=boolean
  Constant4 : Constant
  Filter1 : Subsystem
  Logical Operator2 : Logic  AllPortsSameDT=off  OutDataTypeStr=boolean
  Product3 : Product
  Filtered PV out : Outport
  unfiltered PV OUT : Outport  Port=2
  wires:
  Product3/1 -> unfiltered PV OUT/1, Filter1/1(Signal_in)
  Time/1 -> Compare To Constant1/1
  Constant4/1 -> Logical Operator2/1
  Filter1/1(F_Signal_out) -> Filtered PV out/1
  PV input/1 -> Product3/1
  Logical Operator2/1 -> Product3/2
  Compare To Constant1/1 -> Logical Operator2/2

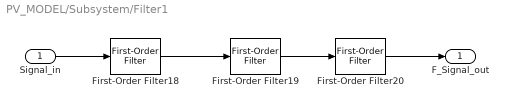
== system PV_MODEL/Subsystem/Filter1 ==
  Signal_in : Inport
  First-Order Filter18 : spsFirstOrderFilterLib/First-Order Filter  FilterType=Lowpass  Tc=1/(2*pi*50)  Ts=0  Initialize=off  Vac_Init=[0, 0, 50]  Vdc_Init=0  PlotResponse=off  FreqRange="[0,  200,  1]"
  First-Order Filter19 : spsFirstOrderFilterLib/First-Order Filter  FilterType=Lowpass  Tc=1/(2*pi*50)  Ts=0  Initialize=off  Vac_Init=[0, 0, 50]  Vdc_Init=0  PlotResponse=off  FreqRange="[0,  200,  1]"
  First-Order Filter20 : spsFirstOrderFilterLib/First-Order Filter  FilterType=Lowpass  Tc=1/(2*pi*50)  Ts=0  Initialize=off  Vac_Init=[0, 0, 50]  Vdc_Init=0  PlotResponse=off  FreqRange="[0,  200,  1]"
  F_Signal_out : Outport
  wires:
  First-Order Filter18/1 -> First-Order Filter19/1
  First-Order Filter20/1 -> F_Signal_out/1
  First-Order Filter19/1 -> First-Order Filter20/1
  Signal_in/1 -> First-Order Filter18/1

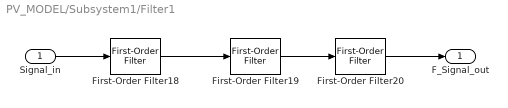
== system PV_MODEL/Subsystem1/Filter1 ==
  Signal_in : Inport
  First-Order Filter18 : spsFirstOrderFilterLib/First-Order Filter  FilterType=Lowpass  Tc=1/(2*pi*50)  Ts=0  Initialize=off  Vac_Init=[0, 0, 50]  Vdc_Init=0  PlotResponse=off  FreqRange="[0,  200,  1]"
  First-Order Filter19 : spsFirstOrderFilterLib/First-Order Filter  FilterType=Lowpass  Tc=1/(2*pi*50)  Ts=0  Initialize=off  Vac_Init=[0, 0, 50]  Vdc_Init=0  PlotResponse=off  FreqRange="[0,  200,  1]"
  First-Order Filter20 : spsFirstOrderFilterLib/First-Order Filter  FilterType=Lowpass  Tc=1/(2*pi*50)  Ts=0  Initialize=off  Vac_Init=[0, 0, 50]  Vdc_Init=0  PlotResponse=off  FreqRange="[0,  200,  1]"
  F_Signal_out : Outport
  wires:
  Signal_in/1 -> First-Order Filter18/1
  First-Order Filter19/1 -> First-Order Filter20/1
  First-Order Filter20/1 -> F_Signal_out/1
  First-Order Filter18/1 -> First-Order Filter19/1

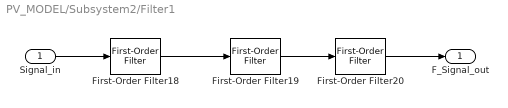
== system PV_MODEL/Subsystem2/Filter1 ==
  Signal_in : Inport
  First-Order Filter18 : spsFirstOrderFilterLib/First-Order Filter  FilterType=Lowpass  Tc=1/(2*pi*50)  Ts=0  Initialize=off  Vac_Init=[0, 0, 50]  Vdc_Init=0  PlotResponse=off  FreqRange="[0,  200,  1]"
  First-Order Filter19 : spsFirstOrderFilterLib/First-Order Filter  FilterType=Lowpass  Tc=1/(2*pi*50)  Ts=0  Initialize=off  Vac_Init=[0, 0, 50]  Vdc_Init=0  PlotResponse=off  FreqRange="[0,  200,  1]"
  First-Order Filter20 : spsFirstOrderFilterLib/First-Order Filter  FilterType=Lowpass  Tc=1/(2*pi*50)  Ts=0  Initialize=off  Vac_Init=[0, 0, 50]  Vdc_Init=0  PlotResponse=off  FreqRange="[0,  200,  1]"
  F_Signal_out : Outport
  wires:
  First-Order Filter18/1 -> First-Order Filter19/1
  First-Order Filter20/1 -> F_Signal_out/1
  First-Order Filter19/1 -> First-Order Filter20/1
  Signal_in/1 -> First-Order Filter18/1

== matlab function PV_MODEL/Variable step P&O MPPT Algorithm ==
  data: I input; V input; Vref output
function Vref = VrefGen(I, V)
% Variable Step Perturb and Observe MPPT Algorithm
% Inputs: I (current), V (voltage)
% Output: Vref (reference voltage)

Vrefmax = 360.6;  % open-circuit voltage for the PV system
Vrefmin = 0.0;    % minimum reference voltage
Vrefinit = 300;   % initial reference voltage
scaling_factor = 0.1; % factor to scale step size based on power gradient
min_step = 0.001; % minimum step size to avoid too small steps
max_step = 0.1;   % maximum step size to avoid instability

persistent Vold Pold Vrefold;

dataType = "double";

if isempty(Vold)
    Vold = 0;
    Pold = 0;
    Vrefold = Vrefinit;
end

P = V * I; % calculating power
dV = V - Vold; % checking for change in voltage
dP = P - Pold; % checking for change in power

% Calculate variable step size based on power gradient
if dV ~= 0
    power_gradient = abs(dP / dV);
    deltaVref = scaling_factor * power_gradient;
    deltaVref = min(max(deltaVref, min_step), max_step); % constrain step size
else
    deltaVref = min_step; % use minimum step if no voltage change
end

%% IMPLEMENTING THE VARIABLE STEP P&O ALGORITHM LOGIC 
if dP ~= 0
    if dP < 0
        if dV < 0
            Vref = Vrefold + deltaVref;
        else
            Vref = Vrefold - deltaVref;
        end
    else
        if dV < 0
            Vref = Vrefold - deltaVref;
        else
            Vref = Vrefold + deltaVref;
        end
    end
else
    Vref = Vrefold;
end

% Boundary check
if Vref >= Vrefmax || Vref <= Vrefmin
    Vref = Vrefold;
end

% Update persistent variables
Vrefold = Vref;
Vold = V;
Pold = P;
end

== matlab function PV_MODEL/Incremental conductance Algorithm ==
  data: I input; V input; Vref output
function Vref = VrefGenIncCond(I, V)
% Variable Step Incremental Conductance MPPT Algorithm
% Inputs: I (current), V (voltage)
% Output: Vref (reference voltage)

Vrefmax = 360.6;  % open-circuit voltage for the PV system
Vrefmin = 0.0;    % minimum reference voltage
Vrefinit = 300;   % initial reference voltage
scaling_factor = 0.1; % factor to scale step size based on power gradient
min_step = 0.001; % minimum step size to avoid too small steps
max_step = 0.1;   % maximum step size to avoid instability

persistent Vold Iold Vrefold;

dataType = "double";

if isempty(Vold)
    Vold = 0;
    Iold = 0;
    Vrefold = Vrefinit;
end

% Calculate incremental and instantaneous conductance
dV = V - Vold;
dI = I - Iold;

% Calculate power for step size adjustment
P = V * I;
Pold = Vold * Iold;
dP = P - Pold;

% Calculate variable step size based on power gradient
if dV ~= 0
    power_gradient = abs(dP / dV);
    deltaVref = scaling_factor * power_gradient;
    deltaVref = min(max(deltaVref, min_step), max_step); % constrain step size
else
    deltaVref = min_step; % use minimum step if no voltage change
end

%% IMPLEMENTING THE INCREMENTAL CONDUCTANCE ALGORITHM LOGIC
if dV == 0
    if dI == 0
        Vref = Vrefold; % At MPP, no change
    elseif dI > 0
        Vref = Vrefold + deltaVref; % Increase voltage
    else
        Vref = Vrefold - deltaVref; % Decrease voltage
    end
else
    conductance = I / V;
    inc_conductance = -dI / dV; % Negative because dI/dV is opposite for MPPT
    if abs(inc_conductance - conductance) < 1e-3 % Tolerance for MPP
        Vref = Vrefold; % At or near MPP
    elseif inc_conductance > conductance
        Vref = Vrefold + deltaVref; % Increase voltage
    else
        Vref = Vrefold - deltaVref; % Decrease voltage
    end
end

% Boundary check
if Vref >= Vrefmax || Vref <= Vrefmin
    Vref = Vrefold;
end

% Update persistent variables
Vrefold = Vref;
Vold = V;
Iold = I;
end

== matlab function PV_MODEL/P&O MPPT Algorithm ==
  data: I input; V input; Vref output
function Vref = VrefGen(I,V)

Vrefmax= 360.6;  %open-circuit voltage for the PV system
Vrefmin=0.0;     %minimum reference voltage
Vrefinit=300;  %initial reference voltage
deltaVref=1; %increment/decrement...
persistent Vold Pold Vrefold;

dataType ="double";

if isempty(Vold)
    Vold=0;
    Pold=0;
    Vrefold=Vrefinit;
end

P=V*I; %calculating power..
dV=V-Vold; %checking for change in voltage
dP=P-Pold; %checking for change in current


%%IMPLEMENTING THE P&O ALGORITHM LOGIC 
if dP ~= 0
    if dP<0
        if dV<0
            Vref=Vrefold+deltaVref;
        else
            Vref=Vrefold-deltaVref;
        end
    else
        if dV<0
            Vref = Vrefold-deltaVref;
        else
            Vref =Vrefold+deltaVref;
        end
    end
else Vref=Vrefold;
end


if Vref >= Vrefmax | Vref <= Vrefmin
    Vref =Vrefold;
end

Vrefold=Vref;
Vold=V;
Pold=P;
end
